simulink library "cntrl_horiz_pos_indi_lib"  (R2018b)
settings: Solver=VariableStepAuto  StartTime=0.0  StopTime=10.0  RelTol=1e-3
undefined symbols (not defined in the file or in its folder): DiscIntNeverNeededParam, horiz_pos_cntrl
libraries: ndi_lib x1, filters_lib x1
settings Model: Creator=Ybeyer  LastModifiedBy=yannic
settings SFSimCC: SimUseLocalCustomCode=off
settings RTWCC: RTWUseLocalCustomCode=off
settings CodeAppCC: StateflowObjectComments=on

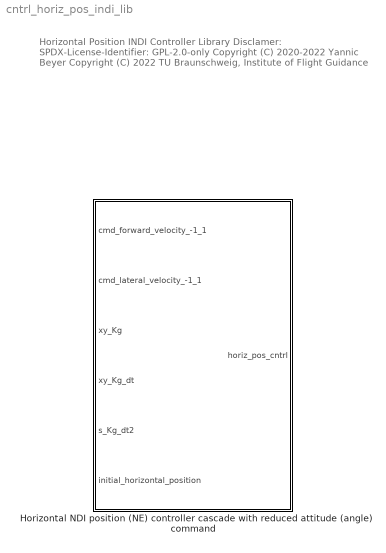
== system cntrl_horiz_pos_indi_lib ==
  note: Horizontal Position INDI Controller Library
      |
      | Disclamer:
      | SPDX-License-Identifier: GPL-2.0-only
      |
      | Copyright (C) 2020-2022 Yannic Beyer
      | Copyright (C) 2022 TU Braunschweig, Institute of Flight Guidance
  Horizontal NDI position (NE) controller cascade with reduced attitude (angle) command : Subsystem  mask{horiz_pos_cntrl=horiz_pos_cntrl, T=0.01}
      mask prompts: horiz_pos_cntrl "horizontal position controller struct"; T "inner loop time constant"
      mask DialogControl DescGroupVar Prompt: Horizontal position controller cascade
      mask DialogControl DescTextVar Prompt: The commanded velocity is filtered and the control error is converted into desired accerlations in x_g and y_g direction. The commanded accelerations are converted into commanded to reduced attitude angles.
      mask DialogControl Control2 Prompt: To initialize a horizontal position controller parameters struct see cntrlHorizPosIndiLoadParams

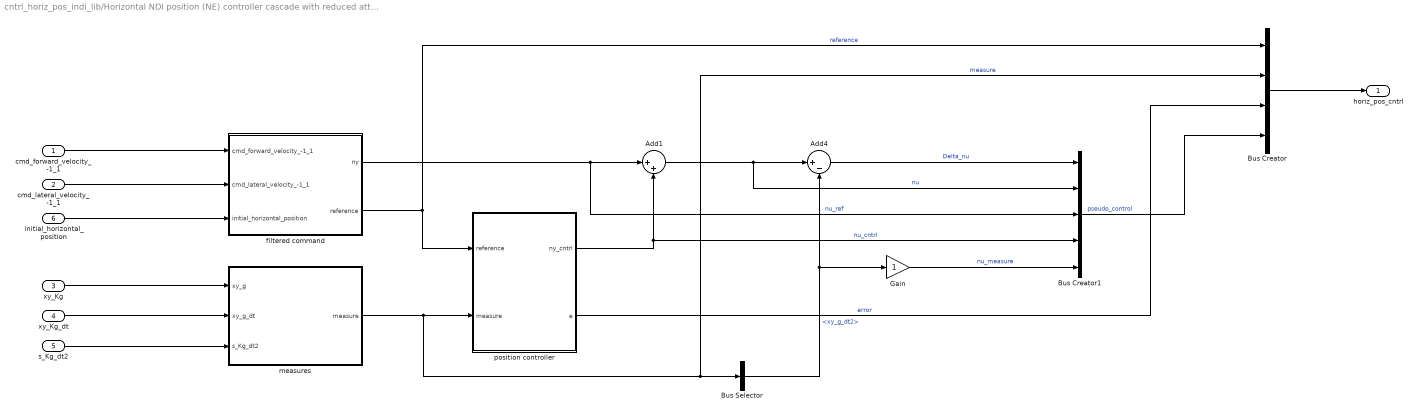
== system cntrl_horiz_pos_indi_lib/Horizontal NDI position (NE) controller cascade with reduced attitude (angle) command ==
  cmd_forward_velocity_-1_1 : Inport
  cmd_lateral_velocity_-1_1 : Inport  Port=2
  xy_Kg : Inport  Port=3
  xy_Kg_dt : Inport  Port=4
  s_Kg_dt2 : Inport  Port=5
  initial_horizontal_position : Inport  Port=6
  Add1 : Sum  Inputs=|++
  Add4 : Sum  Inputs=|+-
  Bus Creator : BusCreator  Inputs=4
  Bus Creator1 : BusCreator  Inputs=5
  Bus Selector : BusSelector  OutputSignals=xy_g_dt2
  Gain : Gain
  filtered command : Subsystem
  measures : Subsystem
  position controller : Subsystem
  horiz_pos_cntrl : Outport
  wires:
  filtered command/1(ny) -> Bus Creator1/3, Add1/1  "nu_ref"
  cmd_forward_velocity_-1_1/1 -> filtered command/1(cmd_forward_velocity_-1_1)
  filtered command/2(reference) -> Bus Creator/1, position controller/1(reference)  "reference"
  initial_horizontal_position/1 -> filtered command/3(initial_horizontal_position)
  position controller/1(ny_cntrl) -> Add1/2, Bus Creator1/4  "nu_cntrl"
  Add1/1 -> Bus Creator1/2, Add4/1  "nu"
  s_Kg_dt2/1 -> measures/3(s_Kg_dt2)
  position controller/2(e) -> Bus Creator/3  "error"
  xy_Kg/1 -> measures/1(xy_g)
  xy_Kg_dt/1 -> measures/2(xy_g_dt)
  cmd_lateral_velocity_-1_1/1 -> filtered command/2(cmd_lateral_velocity_-1_1)
  measures/1(measure) -> Bus Creator/2, Bus Selector/1, position controller/2(measure)  "measure"
  Add4/1 -> Bus Creator1/1  "Delta_nu"
  Bus Selector/1 -> Add4/2, Gain/1  "<xy_g_dt2>"
  Bus Creator1/1 -> Bus Creator/4  "pseudo_control"
  Bus Creator/1 -> horiz_pos_cntrl/1
  Gain/1 -> Bus Creator1/5  "nu_measure"

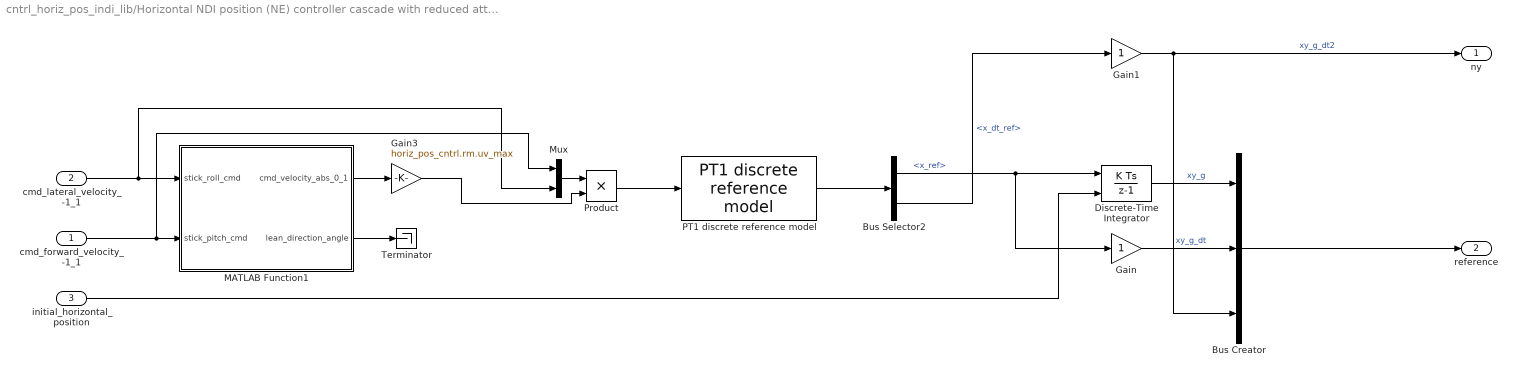
== system cntrl_horiz_pos_indi_lib/Horizontal NDI position (NE) controller cascade with reduced attitude (angle) command/filtered command ==
  cmd_forward_velocity_-1_1 : Inport
  cmd_lateral_velocity_-1_1 : Inport  Port=2
  initial_horizontal_position : Inport  Port=3
  Bus Creator : BusCreator  Inputs=3
  Bus Selector2 : BusSelector  OutputSignals=x_ref,x_dt_ref
  Discrete-Time Integrator : DiscreteIntegrator  InitialConditionSource=external  SampleTime=-1  ICPrevOutput=DiscIntNeverNeededParam  ICPrevScaledInput=DiscIntNeverNeededParam
  Gain : Gain
  Gain1 : Gain
  Gain3 : Gain  Gain=horiz_pos_cntrl.rm.uv_max
  MATLAB Function1 : MATLAB Function  TreatAsAtomicUnit=on
  Mux : Mux  Inputs=2
  PT1 discrete reference model : ndi_lib/PT1 discrete reference model  T=horiz_pos_cntrl.rm.uv_T  x_max=inf  x_min=-inf  x_dt_max=horiz_pos_cntrl.rm.uv_dt_max  x_dt_min=-horiz_pos_cntrl.rm.uv_dt_max  x_init=0
      settings: SourceProductName=LADAC
  Product : Product
  Terminator : Terminator
  ny : Outport
  reference : Outport  Port=2
  wires:
  cmd_forward_velocity_-1_1/1 -> Mux/1, MATLAB Function1/2(stick_pitch_cmd)
  Bus Creator/1 -> reference/1
  PT1 discrete reference model/1 -> Bus Selector2/1
  Discrete-Time Integrator/1 -> Bus Creator/1  "xy_g"
  Bus Selector2/1 -> Gain/1, Discrete-Time Integrator/1  "<x_ref>"
  Bus Selector2/2 -> Gain1/1  "<x_dt_ref>"
  initial_horizontal_position/1 -> Discrete-Time Integrator/2
  cmd_lateral_velocity_-1_1/1 -> Mux/2, MATLAB Function1/1(stick_roll_cmd)
  Gain/1 -> Bus Creator/2  "xy_g_dt"
  Gain1/1 -> ny/1, Bus Creator/3  "xy_g_dt2"
  Mux/1 -> Product/1
  MATLAB Function1/2(lean_direction_angle) -> Terminator/1
  MATLAB Function1/1(cmd_velocity_abs_0_1) -> Gain3/1
  Product/1 -> PT1 discrete reference model/1
  Gain3/1 -> Product/2

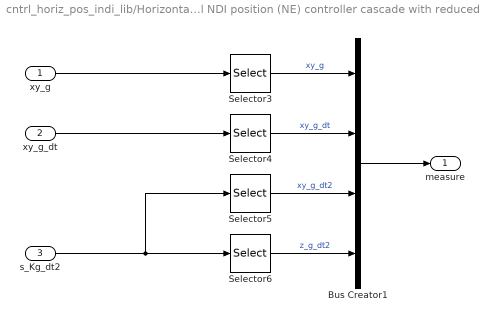
== system cntrl_horiz_pos_indi_lib/Horizontal NDI position (NE) controller cascade with reduced attitude (angle) command/measures ==
  xy_g : Inport
  xy_g_dt : Inport  Port=2
  s_Kg_dt2 : Inport  Port=3
  Bus Creator1 : BusCreator  Inputs=4
  Selector3 : Selector  InputPortWidth=3  IndexOptions=Index vector (dialog)  Indices=[1,2]  OutputSizes=1
  Selector4 : Selector  InputPortWidth=3  IndexOptions=Index vector (dialog)  Indices=[1,2]  OutputSizes=1
  Selector5 : Selector  InputPortWidth=3  IndexOptions=Index vector (dialog)  Indices=[1,2]  OutputSizes=1
  Selector6 : Selector  InputPortWidth=3  IndexOptions=Index vector (dialog)  Indices=3  OutputSizes=1
  measure : Outport
  wires:
  Bus Creator1/1 -> measure/1
  Selector6/1 -> Bus Creator1/4  "z_g_dt2"
  Selector5/1 -> Bus Creator1/3  "xy_g_dt2"
  Selector3/1 -> Bus Creator1/1  "xy_g"
  Selector4/1 -> Bus Creator1/2  "xy_g_dt"
  xy_g/1 -> Selector3/1
  xy_g_dt/1 -> Selector4/1
  s_Kg_dt2/1 -> Selector5/1, Selector6/1

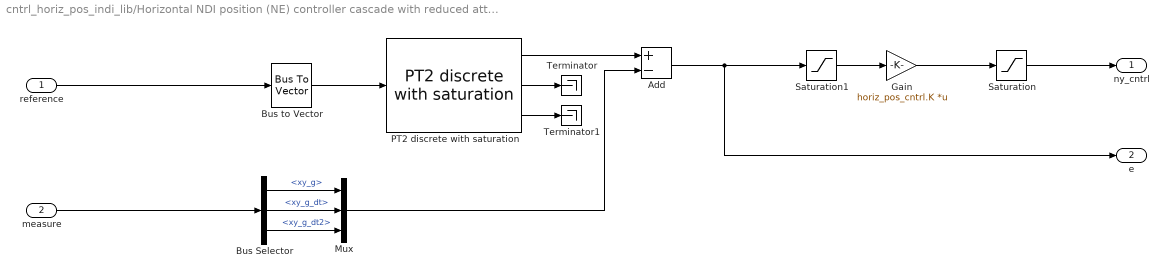
== system cntrl_horiz_pos_indi_lib/Horizontal NDI position (NE) controller cascade with reduced attitude (angle) command/position controller ==
  reference : Inport
  measure : Inport  Port=2
  Add : Sum  Inputs=+-
  Bus Selector : BusSelector  OutputSignals=xy_g,xy_g_dt,xy_g_dt2
  Bus to Vector : BusToVector
  Gain : Gain  Gain=horiz_pos_cntrl.K  Multiplication=Matrix(K*u)
  Mux : Mux  Inputs=3
  PT2 discrete with saturation : filters_lib/PT2 discrete with saturation  omega=2./T  d=1  x_dt2_max=inf  x_dt2_min=-inf  x_dt_max=inf  x_dt_min=-inf  x_max=inf  x_min=-inf  x_init=0  x_dt_init=0
      settings: SourceProductName=LADAC
  Saturation : Saturate  UpperLimit=horiz_pos_cntrl.limits.uv_dt_max  LowerLimit=-horiz_pos_cntrl.limits.uv_dt_max
  Saturation1 : Saturate  UpperLimit=[horiz_pos_cntrl.limits.e_xy_max;1000;1000;1000;1000]  LowerLimit=-[horiz_pos_cntrl.limits.e_xy_max;1000;1000;1000;1000]
  Terminator : Terminator
  Terminator1 : Terminator
  ny_cntrl : Outport
  e : Outport  Port=2
  wires:
  reference/1 -> Bus to Vector/1
  Add/1 -> Saturation1/1, e/1
  Saturation/1 -> ny_cntrl/1
  Saturation1/1 -> Gain/1
  Gain/1 -> Saturation/1
  measure/1 -> Bus Selector/1
  Mux/1 -> Add/2
  Bus Selector/3 -> Mux/3  "<xy_g_dt2>"
  Bus Selector/2 -> Mux/2  "<xy_g_dt>"
  Bus Selector/1 -> Mux/1  "<xy_g>"
  Bus to Vector/1 -> PT2 discrete with saturation/1
  PT2 discrete with saturation/2 -> Terminator/1
  PT2 discrete with saturation/3 -> Terminator1/1
  PT2 discrete with saturation/1 -> Add/1

== matlab function cntrl_horiz_pos_indi_lib/Horizontal NDI position (NE) controller cascade with reduced attitude (angle) command/filtered command/MATLAB Function1 ==
  data: stick_roll_cmd input; cmd_velocity_abs_0_1 output; stick_pitch_cmd input; lean_direction_angle output
function [cmd_velocity_abs_0_1,lean_direction_angle] = fcn(stick_roll_cmd,stick_pitch_cmd)

lean_direction_angle = atan2(stick_roll_cmd,-stick_pitch_cmd);
cmd_velocity_abs_0_1 = sqrt( stick_roll_cmd^2 + stick_pitch_cmd^2 );

end
